simulink model "untitled"  (R2022a)
settings: Solver=VariableStepAuto  StartTime=0.0  StopTime=5  RelTol=1e-3
settings Model: Creator=Todd McKenzie  LastModifiedBy=Todd McKenzie

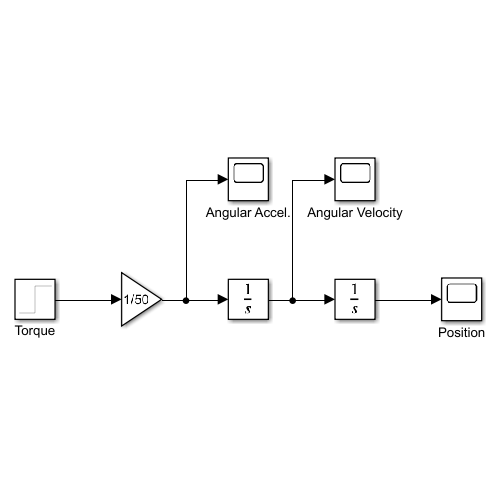
[thumbnail: Simulink's stored preview of the top-level diagram]
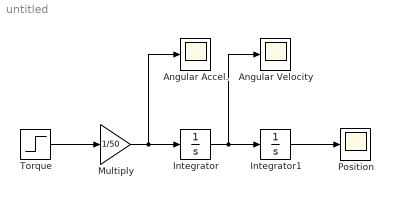
== system untitled ==
  Angular Accel. : Scope
  Angular Velocity : Scope
  Integrator : Integrator
  Integrator1 : Integrator
  Multiply : Gain  Gain=1/50
  Position : Scope
  Torque : Step  Time=0  Before=200  After=200  SampleTime=0
  wires:
  Multiply/1 -> Angular Accel./1, Integrator/1
  Integrator/1 -> Angular Velocity/1, Integrator1/1
  Torque/1 -> Multiply/1
  Integrator1/1 -> Position/1
